simulink model "CSE1_CV3_1Straight"  (Simulink 7.3)
settings: Solver=ode4  StartTime=0.0  StopTime=inf  FixedStep=0.1  RelTol=1e-3
undefined symbols (not defined in the file or in its folder): eta1_0_real, v1_0_real, velocitySatValues1
libraries: simulink x68, dspmtrx3 x24, simulink_extras x23, marine_gnc x5, dspindex x5, dspinverses x4
(part 4 of 6)

== system CSE1_CV3_1Straight/Guidance Systems/Path-following/Line-Of-Sight/Dynamic assigment for sdot ==
  Delta : Inport
  epsilon_n^q : Inport  Port=2
  epsilon_n^s : Inport  Port=3
  epsilon_n : Inport  Port=4
  v_s : Inport  Port=5
  v_s^s : Inport  Port=6
  omega_s : Inport  Port=7
  omega_s^q : Inport  Port=8
  omega_s^s : Inport  Port=9
  v_s^t : Inport  Port=10
  f_s eq : Subsystem
  f_s^q eq : Subsystem
  f_s^s eq : Subsystem
  f_t eq : Subsystem
  f_s : Outport
  f_s^q : Outport  Port=2
  f_s^s : Outport  Port=3
  f_s^t : Outport  Port=4
  wires:
  Delta/1 -> f_s eq/1(Delta), f_s^q eq/1(Delta), f_s^s eq/1(Delta), f_t eq/1(Delta)
  epsilon_n/1 -> f_s eq/2(epsilon_n), f_s^q eq/2(epsilon_n), f_s^s eq/2(epsilon_n), f_t eq/2(epsilon_n)
  v_s/1 -> f_s eq/3(v_s), f_s^q eq/3(v_s), f_s^s eq/3(v_s)
  omega_s/1 -> f_s eq/4(omega_s)
  f_s eq/1(f_s) -> f_s/1
  f_s^q eq/1(f_s^q) -> f_s^q/1
  omega_s^q/1 -> f_s^q eq/4(omega_s^q)
  epsilon_n^q/1 -> f_s^q eq/5(epsilon_n^q)
  f_s^s eq/1(f_s^s) -> f_s^s/1
  omega_s^s/1 -> f_s^s eq/4(omega_s^s)
  epsilon_n^s/1 -> f_s^s eq/5(epsilon_n^s)
  v_s^s/1 -> f_s^s eq/6(v_s^s)
  f_t eq/1(f_t) -> f_s^t/1
  v_s^t/1 -> f_t eq/3(v_s^t)

== system CSE1_CV3_1Straight/Guidance Systems/Path-following/Line-Of-Sight/Gradient update law for sdot ==
  p_d^s^2 : Inport
  p_d^s : Inport  Port=2
  p_d : Inport  Port=3
  q : Inport  Port=4
  my : Inport  Port=5
  |p_d^s| : Inport  Port=6
  Subtract : Sum  Inputs=+-  OutDataType=fixdt(1, 16)  OutScaling=2^-10
  omega_s eq : Subsystem
  omega_s^q eq : Subsystem
  omega_s^s eq : Subsystem
  omega_s : Outport
  omega_s^q : Outport  Port=2
  omega_s^s : Outport  Port=3
  wires:
  p_d^s/1 -> omega_s eq/1(p_d^s), omega_s^q eq/1(p_d^s), omega_s^s eq/1(p_d^s)
  my/1 -> omega_s eq/3(my), omega_s^q eq/2(my), omega_s^s eq/3(my)
  |p_d^s|/1 -> omega_s eq/4(|p_d^s|), omega_s^q eq/3(|p_d^s|), omega_s^s eq/4(|p_d^s|)
  omega_s eq/1(omega_s) -> omega_s/1
  omega_s^q eq/1(omega_s^q) -> omega_s^q/1
  omega_s^s eq/1(omega_s^s) -> omega_s^s/1
  q/1 -> Subtract/1
  p_d/1 -> Subtract/2
  Subtract/1 -> omega_s eq/2(q - p_d), omega_s^s eq/2(q - p_d)
  p_d^s^2/1 -> omega_s^s eq/5(p_d^s^2)

== system CSE1_CV3_1Straight/Guidance Systems/Path-following/Line-Of-Sight/LOS heading ==
  psi_d : Inport
  psi_d^s : Inport  Port=2
  epsilon_n^qs : Inport  Port=3
  epsilon_n^q^2 : Inport  Port=4
  epsilon_n^s^2 : Inport  Port=5
  epsilon_n^q : Inport  Port=6
  epsilon_n^s : Inport  Port=7
  epsilon_n : Inport  Port=8
  psi_d¨^s^2 : Inport  Port=9
  Delta : Inport  Port=10
  psi_los eq : Subsystem
  psi_los^q eq : Subsystem
  psi_los^q^2 eq : Subsystem
  psi_los^qs = psi_los^sq : Subsystem
  psi_los^s eq : Subsystem
  psi_los^s^2 eq : Subsystem
  psi_los^q : Outport
  psi_los^s : Outport  Port=2
  psi_los : Outport  Port=3
  psi_los^qs : Outport  Port=4
  psi_los^q^2 : Outport  Port=5
  psi_los^s^2 : Outport  Port=6
  wires:
  psi_los eq/1(psi_los) -> psi_los/1
  psi_d/1 -> psi_los eq/1(psi_d)
  epsilon_n/1 -> psi_los eq/2(epsilon_n), psi_los^q eq/1(epsilon_n), psi_los^s eq/1(epsilon_n), psi_los^qs = psi_los^sq/1(epsilon_n), psi_los^q^2 eq/1(epsilon_n), psi_los^s^2 eq/1(epsilon_n)
  Delta/1 -> psi_los eq/3(Delta), psi_los^q eq/2(Delta), psi_los^s eq/2(Delta), psi_los^qs = psi_los^sq/2(Delta), psi_los^q^2 eq/2(Delta), psi_los^s^2 eq/2(Delta)
  epsilon_n^q/1 -> psi_los^q eq/3(epsilon_n^q), psi_los^qs = psi_los^sq/4(epsilon_n^q), psi_los^q^2 eq/3(epsilon_n^q)
  psi_los^q eq/1(psi_los^q) -> psi_los^q/1
  psi_los^s eq/1(psi_los^s) -> psi_los^s/1
  psi_d^s/1 -> psi_los^s eq/3(psi_d^s)
  psi_los^qs = psi_los^sq/1(psi_los^qs) -> psi_los^qs/1
  epsilon_n^s/1 -> psi_los^s eq/4(epsilon_n^s), psi_los^qs = psi_los^sq/3(epsilon_n^s), psi_los^s^2 eq/3(epsilon_n^s)
  epsilon_n^qs/1 -> psi_los^qs = psi_los^sq/5(epsilon_n^qs)
  psi_los^q^2 eq/1(psi_los^q^2) -> psi_los^q^2/1
  epsilon_n^q^2/1 -> psi_los^q^2 eq/4(epsilon_n^q^2)
  psi_d¨^s^2/1 -> psi_los^s^2 eq/4(psi_d¨^s^2)
  epsilon_n^s^2/1 -> psi_los^s^2 eq/5(epsilon_n^s^2)
  psi_los^s^2 eq/1(psi_los^s^2) -> psi_los^s^2/1

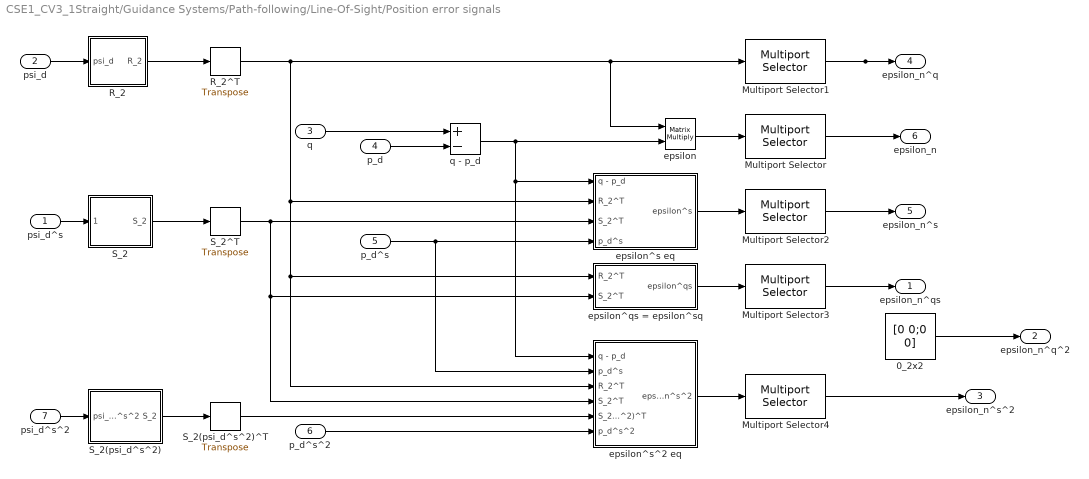
== system CSE1_CV3_1Straight/Guidance Systems/Path-following/Line-Of-Sight/Position error signals ==
  psi_d^s : Inport
  psi_d : Inport  Port=2
  q : Inport  Port=3
  p_d : Inport  Port=4
  p_d^s : Inport  Port=5
  p_d^s^2 : Inport  Port=6
  psi_d^s^2 : Inport  Port=7
  0_2x2 : Constant  Value=[0 0;0 0]  OutDataType=fixdt(1, 16)  OutScaling=2^0
  Multiport Selector{,1..4} (5 alike) : dspindex/Multiport Selector  rowsOrCols=Rows  idxCellArray={2}  idxErrMode=Clip Index
  R_2 : Subsystem  TreatAsAtomicUnit=on
      settings: MinAlgLoopOccurrences=on
  R_2^T : dspmtrx3/Transpose  SystemSampleTime=-1  Hermitian=off  overflowFlag=off
  S_2 : Subsystem  TreatAsAtomicUnit=on
      settings: MinAlgLoopOccurrences=on
  S_2(psi_d^s^2) : Subsystem  TreatAsAtomicUnit=on
      settings: MinAlgLoopOccurrences=on
  S_2(psi_d^s^2)^T : dspmtrx3/Transpose  SystemSampleTime=-1  Hermitian=off  overflowFlag=off
  S_2^T : dspmtrx3/Transpose  SystemSampleTime=-1  Hermitian=off  overflowFlag=off
  epsilon : Product  Multiplication=Matrix(*)  OutDataType=fixdt(1, 16)  OutScaling=2^0  RndMeth=Zero
  epsilon^qs = epsilon^sq : Subsystem
  epsilon^s eq : Subsystem
  epsilon^s^2 eq : Subsystem
  q - p_d : Sum  Inputs=+-  OutDataType=fixdt(1, 16)  OutScaling=2^-10
  epsilon_n^qs : Outport
  epsilon_n^q^2 : Outport  Port=2
  epsilon_n^s^2 : Outport  Port=3
  epsilon_n^q : Outport  Port=4
  epsilon_n^s : Outport  Port=5
  epsilon_n : Outport  Port=6
  wires:
  R_2/1(R_2) -> R_2^T/1
  psi_d/1 -> R_2/1(psi_d)
  q/1 -> q - p_d/1
  p_d/1 -> q - p_d/2
  R_2^T/1 -> epsilon/1, Multiport Selector1/1, epsilon^s eq/2(R_2^T), epsilon^qs = epsilon^sq/1(R_2^T), epsilon^s^2 eq/3(R_2^T)
  q - p_d/1 -> epsilon/2, epsilon^s eq/1(q - p_d), epsilon^s^2 eq/1(q - p_d)
  psi_d^s/1 -> S_2/1(psi_d^s)
  S_2/1(S_2) -> S_2^T/1
  p_d^s/1 -> epsilon^s eq/4(p_d^s), epsilon^s^2 eq/2(p_d^s)
  epsilon^s eq/1(epsilon^s) -> Multiport Selector2/1
  S_2^T/1 -> epsilon^s eq/3(S_2^T), epsilon^qs = epsilon^sq/2(S_2^T), epsilon^s^2 eq/4(S_2^T)
  epsilon^qs = epsilon^sq/1(epsilon^qs) -> Multiport Selector3/1
  0_2x2/1 -> epsilon_n^q^2/1
  epsilon/1 -> Multiport Selector/1
  Multiport Selector/1 -> epsilon_n/1
  Multiport Selector1/1 -> epsilon_n^q/1
  Multiport Selector2/1 -> epsilon_n^s/1
  Multiport Selector3/1 -> epsilon_n^qs/1
  psi_d^s^2/1 -> S_2(psi_d^s^2)/1(psi_d^s^2)
  S_2(psi_d^s^2)/1(S_2) -> S_2(psi_d^s^2)^T/1
  epsilon^s^2 eq/1(epsilon^s^2) -> Multiport Selector4/1
  Multiport Selector4/1 -> epsilon_n^s^2/1
  S_2(psi_d^s^2)^T/1 -> epsilon^s^2 eq/5(S_2(psi_d^s^2)^T)
  p_d^s^2/1 -> epsilon^s^2 eq/6(p_d^s^2)

== system CSE1_CV3_1Straight/Guidance Systems/Path-following/Path/Straight path ==
  s : Inport
  x_1 : Inport  Port=2
  y1 : Inport  Port=3
  x_2 : Inport  Port=4
  y_2 : Inport  Port=5
  0_2x1 : Constant  Value=0  VectorParams1D=off  OutDataType=fixdt(1, 16)  OutScaling=2^0
  Mux1 : Mux  Inputs=2
  p_d eq : Subsystem
  p_d^s eq : Subsystem
  |p_d^s| eq : Subsystem
  p_d : Outport
  p_d^s : Outport  Port=2
  p_d^s^2 : Outport  Port=3
  p_d^s^3 : Outport  Port=4
  |p_d^s| : Outport  Port=5
  wires:
  p_d^s eq/1(p_d^s) -> p_d^s/1, |p_d^s| eq/1(p_d^s)
  |p_d^s| eq/1(|p_d^s|) -> |p_d^s|/1
  s/1 -> p_d eq/1(s)
  x_1/1 -> p_d eq/2(x_1), p_d^s eq/1(x_1)
  y1/1 -> p_d eq/3(y_1), p_d^s eq/2(y_1)
  x_2/1 -> p_d eq/4(x_2), p_d^s eq/3(x_2)
  y_2/1 -> p_d eq/5(y_2), p_d^s eq/4(y_2)
  0_2x1/1 -> Mux1/1, Mux1/2
  Mux1/1 -> p_d^s^2/1, p_d^s^3/1
  p_d eq/1(p_d) -> p_d/1

== system CSE1_CV3_1Straight/Guidance Systems/Path-following/Speed assigment/v_s eq ==
  |p_d^s| : Inport
  u_d : Inport  Port=2
  Divide : Product  Inputs=*/  OutDataType=fixdt(1, 16)  OutScaling=2^-10
  v_s : Outport
  wires:
  Divide/1 -> v_s/1
  u_d/1 -> Divide/1
  |p_d^s|/1 -> Divide/2

== system CSE1_CV3_1Straight/Guidance Systems/Path-following/Speed assigment/v_s^s eq ==
  |p_d^s| : Inport
  u_d : Inport  Port=2
  p_d^s : Inport  Port=3
  p_d^s^2 : Inport  Port=4
  Constant : Constant  Value=3  OutDataType=fixdt(1, 16)  OutScaling=2^0
  Divide : Product  Inputs=*/  OutDataType=fixdt(1, 16)  OutScaling=2^-10
  Gain : Gain  Gain=-1  ParameterDataType=fixdt(1, 16)  ParameterScaling=2^0  OutDataType=fixdt(1, 16)  OutScaling=2^0
  Product : Product  OutDataType=fixdt(1, 16)  OutScaling=2^0  RndMeth=Zero
  Product1 : Product  Multiplication=Matrix(*)  OutDataType=fixdt(1, 16)  OutScaling=2^0  RndMeth=Zero
  p_d^s^T : dspmtrx3/Transpose  SystemSampleTime=-1  Hermitian=off  overflowFlag=off
  |p_d^s|^3 : Math  Operator=pow  OutDataType=fixdt(1, 16)  OutScaling=2^0  SaturateOnIntegerOverflow=on
  v_s^s : Outport
  wires:
  Product/1 -> Gain/1
  p_d^s/1 -> p_d^s^T/1
  p_d^s^T/1 -> Product1/1
  p_d^s^2/1 -> Product1/2
  |p_d^s|/1 -> |p_d^s|^3/1
  Constant/1 -> |p_d^s|^3/2
  Product1/1 -> Divide/1
  |p_d^s|^3/1 -> Divide/2
  Divide/1 -> Product/1
  u_d/1 -> Product/2
  Gain/1 -> v_s^s/1

== system CSE1_CV3_1Straight/Guidance Systems/Path-following/Speed assigment/v_s^t eq ==
  |p_d^s| : Inport
  u_d^t : Inport  Port=2
  Divide : Product  Inputs=*/  OutDataType=fixdt(1, 16)  OutScaling=2^-10
  v_s^t : Outport
  wires:
  Divide/1 -> v_s^t/1
  u_d^t/1 -> Divide/1
  |p_d^s|/1 -> Divide/2

== system CSE1_CV3_1Straight/Plants/Linear Simulator/Linear Vessel Dynamics/D_L ==
  -N_r : Gain  Gain=-1  ParameterDataType=fixdt(1, 16)  ParameterScaling=2^0  OutDataType=fixdt(1, 16)  OutScaling=2^0
  -N_v : Gain  Gain=-1  ParameterDataType=fixdt(1, 16)  ParameterScaling=2^0  OutDataType=fixdt(1, 16)  OutScaling=2^0
  -X_u : Gain  Gain=-1  ParameterDataType=fixdt(1, 16)  ParameterScaling=2^0  OutDataType=fixdt(1, 16)  OutScaling=2^0
  -Y_v : Gain  Gain=-1  ParameterDataType=fixdt(1, 16)  ParameterScaling=2^0  OutDataType=fixdt(1, 16)  OutScaling=2^0
  -Y_vr : Gain  Gain=-1  ParameterDataType=fixdt(1, 16)  ParameterScaling=2^0  OutDataType=fixdt(1, 16)  OutScaling=2^0
  D_L_{12..13,21,31} (4 alike) : Constant  Value=0
  Linear Dampning matrix : Reshape  OutputDimensionality=Customize  OutputDimensions=[3,3]
  Mux : Mux  Inputs=9
  N_r : Constant  Value=-1.900
  N_v : Constant  Value=0.18140
  X_u : Constant  Value=-0.59739
  Y_r : Constant  Value=-7.250
  Y_v : Constant  Value=-3.50625
  D_L : Outport
  wires:
  X_u/1 -> -X_u/1
  Mux/1 -> Linear Dampning matrix/1
  Linear Dampning matrix/1 -> D_L/1
  Y_v/1 -> -Y_v/1
  N_v/1 -> -N_v/1
  Y_r/1 -> -Y_vr/1
  N_r/1 -> -N_r/1
  -X_u/1 -> Mux/1
  D_L_21/1 -> Mux/2
  D_L_31/1 -> Mux/3
  D_L_12/1 -> Mux/4
  -Y_v/1 -> Mux/5
  -N_v/1 -> Mux/6
  D_L_13/1 -> Mux/7
  -Y_vr/1 -> Mux/8
  -N_r/1 -> Mux/9

== system CSE1_CV3_1Straight/Plants/Linear Simulator/Linear Vessel Dynamics/Initial eta ==
  Mux : Mux  Inputs=3
  psi_0 : Constant  Value=0  OutDataType=fixdt(1, 16)  OutScaling=2^0
  x_0 : Constant  Value=0  OutDataType=fixdt(1, 16)  OutScaling=2^0
  y_0 : Constant  Value=0  OutDataType=fixdt(1, 16)  OutScaling=2^0
  eta_0 : Outport  OutDataType=fixdt(1, 16)  OutScaling=2^0
  wires:
  x_0/1 -> Mux/1
  y_0/1 -> Mux/2
  psi_0/1 -> Mux/3
  Mux/1 -> eta_0/1

== system CSE1_CV3_1Straight/Plants/Linear Simulator/Linear Vessel Dynamics/Initial nu ==
  Mux : Mux  Inputs=3
  r_0 : Constant  Value=0  OutDataType=fixdt(1, 16)  OutScaling=2^0
  u_0 : Constant  Value=0  OutDataType=fixdt(1, 16)  OutScaling=2^0
  v_0 : Constant  Value=0  OutDataType=fixdt(1, 16)  OutScaling=2^0
  nu_0 : Outport  OutDataType=fixdt(1, 16)  OutScaling=2^0
  wires:
  u_0/1 -> Mux/1
  v_0/1 -> Mux/2
  r_0/1 -> Mux/3
  Mux/1 -> nu_0/1

== system CSE1_CV3_1Straight/Plants/Linear Simulator/Linear Vessel Dynamics/M_inv ==
  I_z : Constant  Value=1.760
  Inverse : Product  Inputs=/  Multiplication=Matrix(*)
  M : Reshape  OutputDimensionality=Customize  OutputDimensions=[3,3]
  M_{11,22..23,32..33} (5 alike) : Sum  Inputs=+-
  M_{12..13,21,31} (4 alike) : Constant  Value=0
  Mux : Mux  Inputs=9
  N_rdot : Constant  Value=-1.0
  N_vdot : Constant  Value=-0.0
  X_udot : Constant  Value=-2.0
  Y_rdot : Constant  Value=0.0
  Y_vdot : Constant  Value=-10.0
  m : Constant  Value=17.6
  m x_g : Product  RndMeth=Zero
  x_g : Constant  Value=0.03
  M_inv : Outport
  wires:
  m/1 -> M_11/1, M_22/1, m x_g/1
  X_udot/1 -> M_11/2
  Y_vdot/1 -> M_22/2
  x_g/1 -> m x_g/2
  m x_g/1 -> M_32/1, M_23/1
  N_vdot/1 -> M_32/2
  Y_rdot/1 -> M_23/2
  I_z/1 -> M_33/1
  N_rdot/1 -> M_33/2
  Inverse/1 -> M_inv/1
  M_11/1 -> Mux/1
  M_21/1 -> Mux/2
  M_31/1 -> Mux/3
  M_12/1 -> Mux/4
  M_22/1 -> Mux/5
  M_32/1 -> Mux/6
  M_13/1 -> Mux/7
  M_23/1 -> Mux/8
  M_33/1 -> Mux/9
  Mux/1 -> M/1
  M/1 -> Inverse/1

== system CSE1_CV3_1Straight/Plants/Linear Simulator/Linear Vessel Dynamics/R(psi) ==
  psi : Inport
  Mux : Mux  Inputs=9
  R(psi) : Reshape  OutputDimensionality=Customize  OutputDimensions=[3,3]
  R11 : Fcn  Expr=cos(u(1))
  R12 : Fcn  Expr=-1*sin(u(1))
  R{13,23,31..32} (4 alike) : Constant  Value=0
  R21 : Fcn  Expr=sin(u(1))
  R22 : Fcn  Expr=cos(u(1))
  R33 : Constant
  R : Outport
  wires:
  R(psi)/1 -> R/1
  Mux/1 -> R(psi)/1
  psi/1 -> R11/1, R21/1, R12/1, R22/1
  R11/1 -> Mux/1
  R21/1 -> Mux/2
  R31/1 -> Mux/3
  R12/1 -> Mux/4
  R22/1 -> Mux/5
  R32/1 -> Mux/6
  R13/1 -> Mux/7
  R33/1 -> Mux/9
  R23/1 -> Mux/8

== system CSE1_CV3_1Straight/Control Systems/DP control/Thruster allocation/f_act to u_act/f_1 to u_1 ==
  note: If < 0: control input is 1
      | if = 0 control input is 2
      | if > 0: control input is 3
  note: Check if the input value is less, equal or greater then zero
  note: The mapping is divided into 3 parts:
      | negative, zero and positive
  f_1 : Inport
  Gain : Gain  Gain=2  ParameterDataType=fixdt(1, 16)  ParameterScaling=2^0  OutDataType=fixdt(1, 16)  OutScaling=2^0
  Gain1 : Gain  Gain=3  ParameterDataType=fixdt(1, 16)  ParameterScaling=2^0  OutDataType=fixdt(1, 16)  OutScaling=2^0
  If < 0 : simulink/Logic and Bit Operations/Compare To Constant  SystemSampleTime=-1  relop=<  const=0  LogicOutDataTypeMode=uint8
  If > 0 : simulink/Logic and Bit Operations/Compare To Constant  SystemSampleTime=-1  relop=>  const=0  LogicOutDataTypeMode=uint8
  Multiport Switch : MultiPortSwitch  OutDataType=fixdt(1, 16)  OutScaling=2^0
  Sum : Sum  Inputs=+++  OutDataType=fixdt(1, 16)  OutScaling=2^0
  f_1 < 0 : Lookup  InputValues=|  Table=|  LookUpMeth=Interpolation-Use End Values  OutDataType=fixdt(1, 16)  OutScaling=2^0
      InputValues=|
      | [-1.324
      | -1.169
      | -0.919
      | -0.703
      | -0.535
      | -0.292
      | -0.165
      | -0.060
      | 0]
      Table=|
      | [-1.0000
      |    -0.9000
      |    -0.8000
      |    -0.7000
      |    -0.6000
      |    -0.5000
      |    -0.4000
      |    -0.3000
      |    -0.2089]
  f_1 = 0 : Constant  Value=0  OutDataType=fixdt(1, 16)  OutScaling=2^0
  f_1 > 0 : Lookup  InputValues=|  Table=|  LookUpMeth=Interpolation-Use End Values  OutDataType=fixdt(1, 16)  OutScaling=2^0
      InputValues=|
      | [0
      |     0.0510
      |     0.1530
      |     0.3080
      |     0.4800
      |     0.6630
      |     0.9110
      |     1.0570
      |     1.2210
      |     1.3740]
      Table=|
      | [0.0500
      |     0.1000
      |     0.2000
      |     0.3000
      |     0.4000
      |     0.5000
      |     0.6000
      |     0.7000
      |     0.8000
      |     0.9000]
  if == 0 : simulink/Logic and Bit Operations/Compare To Zero  SystemSampleTime=-1  relop===  LogicOutDataTypeMode=uint8
  u_1 : Outport
  wires:
  Multiport Switch/1 -> u_1/1
  Gain1/1 -> Sum/3
  Gain/1 -> Sum/2
  Sum/1 -> Multiport Switch/1
  If > 0/1 -> Gain1/1
  if == 0/1 -> Gain/1
  If < 0/1 -> Sum/1
  f_1/1 -> f_1 < 0/1, f_1 > 0/1, If < 0/1, if == 0/1, If > 0/1
  f_1 < 0/1 -> Multiport Switch/2
  f_1 = 0/1 -> Multiport Switch/3
  f_1 > 0/1 -> Multiport Switch/4

== system CSE1_CV3_1Straight/Control Systems/DP control/Thruster allocation/f_act to u_act/f_2 to u_2 ==
  note: If < 0: control input is 1
      | if = 0 control input is 2
      | if > 0: control input is 3
  note: Check if the input value is less, equal or greater then zero
  note: The mapping is divided into 3 parts:
      | Negative, zero and positive
  f_2 : Inport
  Gain : Gain  Gain=2  ParameterDataType=fixdt(1, 16)  ParameterScaling=2^0  OutDataType=fixdt(1, 16)  OutScaling=2^0
  Gain1 : Gain  Gain=3  ParameterDataType=fixdt(1, 16)  ParameterScaling=2^0  OutDataType=fixdt(1, 16)  OutScaling=2^0
  If < 0 : simulink/Logic and Bit Operations/Compare To Constant  SystemSampleTime=-1  relop=<  const=0  LogicOutDataTypeMode=uint8
  If > 0 : simulink/Logic and Bit Operations/Compare To Constant  SystemSampleTime=-1  relop=>  const=0  LogicOutDataTypeMode=uint8
  Multiport Switch : MultiPortSwitch  OutDataType=fixdt(1, 16)  OutScaling=2^0
  Sum : Sum  Inputs=+++  OutDataType=fixdt(1, 16)  OutScaling=2^0
  f_2 < 0 : Lookup  InputValues=|  Table=|  LookUpMeth=Interpolation-Use End Values  OutDataType=fixdt(1, 16)  OutScaling=2^0
      InputValues=|
      | [-0.766
      | -0.649
      | -0.522
      | -0.411
      | -0.323
      | -0.246
      | -0.156
      | -0.075
      | -0.018
      | -0.006
      | 0]
      Table=|
      | [-1.0000
      |    -0.9000
      |    -0.8000
      |    -0.7000
      |    -0.6000
      |    -0.5000
      |    -0.4000
      |    -0.3000
      |    -0.2000
      |    -0.1000
      |    -0.0466]
  f_2 = 0 : Constant  Value=0  OutDataType=fixdt(1, 16)  OutScaling=2^0
  f_2 > 0 : Lookup  InputValues=|  Table=|  LookUpMeth=Interpolation-Use End Values  OutDataType=fixdt(1, 16)  OutScaling=2^0
      InputValues=|
      | [0.000
      | 0.052
      | 0.207
      | 0.331
      | 0.509
      | 0.689
      | 0.829
      | 0.961
      | 1.079
      | 1.120
      | ]
      Table=|
      | [0.1665
      |     0.2000
      |     0.3000
      |     0.4000
      |     0.5000
      |     0.6000
      |     0.7000
      |     0.8000
      |     0.9000
      |     1.0000]
  if == 0 : simulink/Logic and Bit Operations/Compare To Zero  SystemSampleTime=-1  relop===  LogicOutDataTypeMode=uint8
  u_2 : Outport
  wires:
  f_2 > 0/1 -> Multiport Switch/4
  f_2 = 0/1 -> Multiport Switch/3
  f_2 < 0/1 -> Multiport Switch/2
  f_2/1 -> If > 0/1, if == 0/1, If < 0/1, f_2 > 0/1, f_2 < 0/1
  If < 0/1 -> Sum/1
  if == 0/1 -> Gain/1
  If > 0/1 -> Gain1/1
  Sum/1 -> Multiport Switch/1
  Gain/1 -> Sum/2
  Gain1/1 -> Sum/3
  Multiport Switch/1 -> u_2/1

== system CSE1_CV3_1Straight/Control Systems/DP control/Thruster allocation/f_act to u_act/f_3 to u_3 ==
  note: If < 0: control input is 1
      | if = 0 control input is 2
      | if > 0: control input is 3
  note: Check if the input value is less, equal or greater then zero
  note: The mapping is divided into 3 parts:
      | Negative, zero and positive
  f_3 : Inport
  Gain : Gain  Gain=2  ParameterDataType=fixdt(1, 16)  ParameterScaling=2^0  OutDataType=fixdt(1, 16)  OutScaling=2^0
  Gain1 : Gain  Gain=3  ParameterDataType=fixdt(1, 16)  ParameterScaling=2^0  OutDataType=fixdt(1, 16)  OutScaling=2^0
  If < 0 : simulink/Logic and Bit Operations/Compare To Constant  SystemSampleTime=-1  relop=<  const=0  LogicOutDataTypeMode=uint8
  If > 0 : simulink/Logic and Bit Operations/Compare To Constant  SystemSampleTime=-1  relop=>  const=0  LogicOutDataTypeMode=uint8
  Multiport Switch : MultiPortSwitch  OutDataType=fixdt(1, 16)  OutScaling=2^0
  Sum : Sum  Inputs=+++  OutDataType=fixdt(1, 16)  OutScaling=2^0
  f_3 < 0 : Lookup  InputValues=|  Table=|  LookUpMeth=Interpolation-Use End Values  OutDataType=fixdt(1, 16)  OutScaling=2^0
      InputValues=|
      | [-1.291
      | -1.088
      | -0.885
      | -0.618
      | -0.403
      | -0.211
      | -0.034
      | 0.000]
      Table=|
      | [-0.9000
      |    -0.8000
      |    -0.7000
      |    -0.6000
      |    -0.5000
      |    -0.4000
      |    -0.3000
      |    -0.2809]
  f_3 = 0 : Constant  Value=0  OutDataType=fixdt(1, 16)  OutScaling=2^0
  f_3 > 0 : Lookup  InputValues=|  Table=|  LookUpMeth=Interpolation-Use End Values  OutDataType=fixdt(1, 16)  OutScaling=2^0
      InputValues=|
      | [0.000
      | 0.014
      | 0.040
      | 0.147
      | 0.302
      | 0.494
      | 0.680
      | 0.968
      | 1.111
      | 1.289
      | 1.339]
      Table=|
      | [0.0452
      |     0.1000
      |     0.2000
      |     0.3000
      |     0.4000
      |     0.5000
      |     0.6000
      |     0.7000
      |     0.8000
      |     0.9000
      |     1.0000
      | ]
  if == 0 : simulink/Logic and Bit Operations/Compare To Zero  SystemSampleTime=-1  relop===  LogicOutDataTypeMode=uint8
  u_3 : Outport
  wires:
  Multiport Switch/1 -> u_3/1
  Gain1/1 -> Sum/3
  Gain/1 -> Sum/2
  Sum/1 -> Multiport Switch/1
  If > 0/1 -> Gain1/1
  if == 0/1 -> Gain/1
  If < 0/1 -> Sum/1
  f_3/1 -> f_3 < 0/1, f_3 > 0/1, If < 0/1, if == 0/1, If > 0/1
  f_3 < 0/1 -> Multiport Switch/2
  f_3 = 0/1 -> Multiport Switch/3
  f_3 > 0/1 -> Multiport Switch/4

== system CSE1_CV3_1Straight/Control Systems/DP control/Thruster allocation/f_act to u_act/f_4 to u_4 ==
  note: If < 0: control input is 1
      | if = 0 control input is 2
      | if > 0: control input is 3
  note: Check if the input value is less, equal or greater then zero
  note: The mapping is divided into 3 parts:
      | Negative, zero and positive
  f_4 : Inport
  Gain : Gain  Gain=2  ParameterDataType=fixdt(1, 16)  ParameterScaling=2^0  OutDataType=fixdt(1, 16)  OutScaling=2^0
  Gain1 : Gain  Gain=3  ParameterDataType=fixdt(1, 16)  ParameterScaling=2^0  OutDataType=fixdt(1, 16)  OutScaling=2^0
  If < 0 : simulink/Logic and Bit Operations/Compare To Constant  SystemSampleTime=-1  relop=<  const=0  LogicOutDataTypeMode=uint8
  If > 0 : simulink/Logic and Bit Operations/Compare To Constant  SystemSampleTime=-1  relop=>  const=0  LogicOutDataTypeMode=uint8
  Multiport Switch : MultiPortSwitch  OutDataType=fixdt(1, 16)  OutScaling=2^0
  Sum : Sum  Inputs=+++  OutDataType=fixdt(1, 16)  OutScaling=2^0
  f_4 < 0 : Lookup  InputValues=|  Table=|  LookUpMeth=Interpolation-Use End Values  OutDataType=fixdt(1, 16)  OutScaling=2^0
      InputValues=|
      | [-1.249
      | -1.225
      | -1.094
      | -0.896
      | -0.696
      | -0.502
      | -0.314
      | -0.169
      | -0.042
      | 0.000]
      Table=|
      | [-0.9000
      |    -0.8000
      |    -0.7000
      |    -0.6000
      |    -0.5000
      |    -0.4000
      |    -0.3000
      |    -0.2000
      |    -0.1000
      |    -0.0674]
  f_4 = 0 : Constant  Value=0  OutDataType=fixdt(1, 16)  OutScaling=2^0
  f_4 > 0 : Lookup  InputValues=|  Table=|  LookUpMeth=Interpolation-Use End Values  OutDataType=fixdt(1, 16)  OutScaling=2^0
      InputValues=|
      | [0.000
      | 0.063
      | 0.107
      | 0.274
      | 0.441
      | 0.599
      | 0.731]
      Table=|
      | [0.3588
      |     0.5000
      |     0.6000
      |     0.7000
      |     0.8000
      |     0.9000
      |     1.0000]
  if == 0 : simulink/Logic and Bit Operations/Compare To Zero  SystemSampleTime=-1  relop===  LogicOutDataTypeMode=uint8
  u_4 : Outport
  wires:
  f_4 > 0/1 -> Multiport Switch/4
  f_4 = 0/1 -> Multiport Switch/3
  f_4 < 0/1 -> Multiport Switch/2
  f_4/1 -> If > 0/1, if == 0/1, If < 0/1, f_4 > 0/1, f_4 < 0/1
  If < 0/1 -> Sum/1
  if == 0/1 -> Gain/1
  If > 0/1 -> Gain1/1
  Sum/1 -> Multiport Switch/1
  Gain/1 -> Sum/2
  Gain1/1 -> Sum/3
  Multiport Switch/1 -> u_4/1

== system CSE1_CV3_1Straight/Control Systems/DP control/Thruster allocation/f_act to u_act/f_5 to u_5 ==
  note: The mapping is divided into 3 parts:
      | Negative, zero and positive
  note: Check if the input value is less, equal or greater then zero
  note: If < 0: control input is 1
      | if = 0 control input is 2
      | if > 0: control input is 3
  f_5 : Inport
  Gain : Gain  Gain=2  ParameterDataType=fixdt(1, 16)  ParameterScaling=2^0  OutDataType=fixdt(1, 16)  OutScaling=2^0
  Gain1 : Gain  Gain=3  ParameterDataType=fixdt(1, 16)  ParameterScaling=2^0  OutDataType=fixdt(1, 16)  OutScaling=2^0
  If < 0 : simulink/Logic and Bit Operations/Compare To Constant  SystemSampleTime=-1  relop=<  const=0  LogicOutDataTypeMode=uint8
  If > 0 : simulink/Logic and Bit Operations/Compare To Constant  SystemSampleTime=-1  relop=>  const=0  LogicOutDataTypeMode=uint8
  Multiport Switch : MultiPortSwitch  OutDataType=fixdt(1, 16)  OutScaling=2^0
  Sum : Sum  Inputs=+++  OutDataType=fixdt(1, 16)  OutScaling=2^0
  f_5 < 0 : Lookup  InputValues=|  Table=|  LookUpMeth=Interpolation-Use End Values  OutDataType=fixdt(1, 16)  OutScaling=2^0
      InputValues=|
      | [-1.2630
      |    -1.0309
      |    -0.3808]
      Table=|
      | [-0.3000
      |    -0.2000
      |    -0.1000]
  f_5 = 0 : Constant  Value=0  OutDataType=fixdt(1, 16)  OutScaling=2^0
  f_5 > 0 : Lookup  InputValues=|  Table=|  LookUpMeth=Interpolation-Use End Values  OutDataType=fixdt(1, 16)  OutScaling=2^0
      InputValues=|
      | [0.3480
      |     0.8290
      |     1.0930]
      Table=|
      | [0.1000
      |     0.2000
      |     0.3000]
  if == 0 : simulink/Logic and Bit Operations/Compare To Zero  SystemSampleTime=-1  relop===  LogicOutDataTypeMode=uint8
  u_5 : Outport
  wires:
  Multiport Switch/1 -> u_5/1
  Gain1/1 -> Sum/3
  Gain/1 -> Sum/2
  Sum/1 -> Multiport Switch/1
  If > 0/1 -> Gain1/1
  if == 0/1 -> Gain/1
  If < 0/1 -> Sum/1
  f_5/1 -> f_5 < 0/1, f_5 > 0/1, If < 0/1, if == 0/1, If > 0/1
  f_5 < 0/1 -> Multiport Switch/2
  f_5 = 0/1 -> Multiport Switch/3
  f_5 > 0/1 -> Multiport Switch/4

== system CSE1_CV3_1Straight/Control Systems/DP control/Thruster allocation/tau to f_act/T_e ==
  -l_x1 : Gain  Gain=-1
  -l_x2 : Gain  Gain=-1
  -l_y2 : Gain  Gain=-1
  3x5 : Reshape  OutputDimensionality=Customize  OutputDimensions=[3,5]
  Mux : Mux  Inputs=15
  T_e{11,13,22,24..25} (5 alike) : Constant
  T_e{12,14..15,21,23} (5 alike) : Constant  Value=0
  l_x1 : Constant  Value=0.45
  l_x2 : Constant  Value=0.45
  l_x3 : Constant  Value=0.385
  l_y1 : Constant  Value=0.055
  l_y2 : Constant  Value=0.055
  T_e : Outport
  wires:
  l_x3/1 -> Mux/15
  T_e25/1 -> Mux/14
  T_e15/1 -> Mux/13
  -l_x2/1 -> Mux/12
  -l_y2/1 -> Mux/9
  -l_x1/1 -> Mux/6
  l_x2/1 -> -l_x2/1
  T_e24/1 -> Mux/11
  T_e14/1 -> Mux/10
  l_y2/1 -> -l_y2/1
  T_e23/1 -> Mux/8
  T_e13/1 -> Mux/7
  l_x1/1 -> -l_x1/1
  T_e22/1 -> Mux/5
  T_e12/1 -> Mux/4
  l_y1/1 -> Mux/3
  T_e21/1 -> Mux/2
  T_e11/1 -> Mux/1
  3x5/1 -> T_e/1
  Mux/1 -> 3x5/1

== system CSE1_CV3_1Straight/Control Systems/LgV design 2/Thruster allocation/f_act to u_act/f_1 to u_1 ==
  note: If < 0: control input is 1
      | if = 0 control input is 2
      | if > 0: control input is 3
  note: Check if the input value is less, equal or greater then zero
  note: The mapping is divided into 3 parts:
      | negative, zero and positive
  f_1 : Inport
  Gain : Gain  Gain=2  ParameterDataType=fixdt(1, 16)  ParameterScaling=2^0  OutDataType=fixdt(1, 16)  OutScaling=2^0
  Gain1 : Gain  Gain=3  ParameterDataType=fixdt(1, 16)  ParameterScaling=2^0  OutDataType=fixdt(1, 16)  OutScaling=2^0
  If < 0 : simulink/Logic and Bit Operations/Compare To Constant  SystemSampleTime=-1  relop=<  const=0  LogicOutDataTypeMode=uint8
  If > 0 : simulink/Logic and Bit Operations/Compare To Constant  SystemSampleTime=-1  relop=>  const=0  LogicOutDataTypeMode=uint8
  Multiport Switch : MultiPortSwitch  OutDataType=fixdt(1, 16)  OutScaling=2^0
  Sum : Sum  Inputs=+++  OutDataType=fixdt(1, 16)  OutScaling=2^0
  f_1 < 0 : Lookup  InputValues=|  Table=|  LookUpMeth=Interpolation-Use End Values  OutDataType=fixdt(1, 16)  OutScaling=2^0
      InputValues=|
      | [-1.324
      | -1.169
      | -0.919
      | -0.703
      | -0.535
      | -0.292
      | -0.165
      | -0.060
      | 0]
      Table=|
      | [-1.0000
      |    -0.9000
      |    -0.8000
      |    -0.7000
      |    -0.6000
      |    -0.5000
      |    -0.4000
      |    -0.3000
      |    -0.2089]
  f_1 = 0 : Constant  Value=0  OutDataType=fixdt(1, 16)  OutScaling=2^0
  f_1 > 0 : Lookup  InputValues=|  Table=|  LookUpMeth=Interpolation-Use End Values  OutDataType=fixdt(1, 16)  OutScaling=2^0
      InputValues=|
      | [0
      |     0.0510
      |     0.1530
      |     0.3080
      |     0.4800
      |     0.6630
      |     0.9110
      |     1.0570
      |     1.2210
      |     1.3740]
      Table=|
      | [0.0500
      |     0.1000
      |     0.2000
      |     0.3000
      |     0.4000
      |     0.5000
      |     0.6000
      |     0.7000
      |     0.8000
      |     0.9000]
  if == 0 : simulink/Logic and Bit Operations/Compare To Zero  SystemSampleTime=-1  relop===  LogicOutDataTypeMode=uint8
  u_1 : Outport
  wires:
  Multiport Switch/1 -> u_1/1
  Gain1/1 -> Sum/3
  Gain/1 -> Sum/2
  Sum/1 -> Multiport Switch/1
  If > 0/1 -> Gain1/1
  if == 0/1 -> Gain/1
  If < 0/1 -> Sum/1
  f_1/1 -> f_1 < 0/1, f_1 > 0/1, If < 0/1, if == 0/1, If > 0/1
  f_1 < 0/1 -> Multiport Switch/2
  f_1 = 0/1 -> Multiport Switch/3
  f_1 > 0/1 -> Multiport Switch/4

== system CSE1_CV3_1Straight/Control Systems/LgV design 2/Thruster allocation/f_act to u_act/f_2 to u_2 ==
  note: If < 0: control input is 1
      | if = 0 control input is 2
      | if > 0: control input is 3
  note: Check if the input value is less, equal or greater then zero
  note: The mapping is divided into 3 parts:
      | Negative, zero and positive
  f_2 : Inport
  Gain : Gain  Gain=2  ParameterDataType=fixdt(1, 16)  ParameterScaling=2^0  OutDataType=fixdt(1, 16)  OutScaling=2^0
  Gain1 : Gain  Gain=3  ParameterDataType=fixdt(1, 16)  ParameterScaling=2^0  OutDataType=fixdt(1, 16)  OutScaling=2^0
  If < 0 : simulink/Logic and Bit Operations/Compare To Constant  SystemSampleTime=-1  relop=<  const=0  LogicOutDataTypeMode=uint8
  If > 0 : simulink/Logic and Bit Operations/Compare To Constant  SystemSampleTime=-1  relop=>  const=0  LogicOutDataTypeMode=uint8
  Multiport Switch : MultiPortSwitch  OutDataType=fixdt(1, 16)  OutScaling=2^0
  Sum : Sum  Inputs=+++  OutDataType=fixdt(1, 16)  OutScaling=2^0
  f_2 < 0 : Lookup  InputValues=|  Table=|  LookUpMeth=Interpolation-Use End Values  OutDataType=fixdt(1, 16)  OutScaling=2^0
      InputValues=|
      | [-0.766
      | -0.649
      | -0.522
      | -0.411
      | -0.323
      | -0.246
      | -0.156
      | -0.075
      | -0.018
      | -0.006
      | 0]
      Table=|
      | [-1.0000
      |    -0.9000
      |    -0.8000
      |    -0.7000
      |    -0.6000
      |    -0.5000
      |    -0.4000
      |    -0.3000
      |    -0.2000
      |    -0.1000
      |    -0.0466]
  f_2 = 0 : Constant  Value=0  OutDataType=fixdt(1, 16)  OutScaling=2^0
  f_2 > 0 : Lookup  InputValues=|  Table=|  LookUpMeth=Interpolation-Use End Values  OutDataType=fixdt(1, 16)  OutScaling=2^0
      InputValues=|
      | [0.000
      | 0.052
      | 0.207
      | 0.331
      | 0.509
      | 0.689
      | 0.829
      | 0.961
      | 1.079
      | 1.120
      | ]
      Table=|
      | [0.1665
      |     0.2000
      |     0.3000
      |     0.4000
      |     0.5000
      |     0.6000
      |     0.7000
      |     0.8000
      |     0.9000
      |     1.0000]
  if == 0 : simulink/Logic and Bit Operations/Compare To Zero  SystemSampleTime=-1  relop===  LogicOutDataTypeMode=uint8
  u_2 : Outport
  wires:
  f_2 > 0/1 -> Multiport Switch/4
  f_2 = 0/1 -> Multiport Switch/3
  f_2 < 0/1 -> Multiport Switch/2
  f_2/1 -> If > 0/1, if == 0/1, If < 0/1, f_2 > 0/1, f_2 < 0/1
  If < 0/1 -> Sum/1
  if == 0/1 -> Gain/1
  If > 0/1 -> Gain1/1
  Sum/1 -> Multiport Switch/1
  Gain/1 -> Sum/2
  Gain1/1 -> Sum/3
  Multiport Switch/1 -> u_2/1

== system CSE1_CV3_1Straight/Control Systems/LgV design 2/Thruster allocation/f_act to u_act/f_3 to u_3 ==
  note: If < 0: control input is 1
      | if = 0 control input is 2
      | if > 0: control input is 3
  note: Check if the input value is less, equal or greater then zero
  note: The mapping is divided into 3 parts:
      | Negative, zero and positive
  f_3 : Inport
  Gain : Gain  Gain=2  ParameterDataType=fixdt(1, 16)  ParameterScaling=2^0  OutDataType=fixdt(1, 16)  OutScaling=2^0
  Gain1 : Gain  Gain=3  ParameterDataType=fixdt(1, 16)  ParameterScaling=2^0  OutDataType=fixdt(1, 16)  OutScaling=2^0
  If < 0 : simulink/Logic and Bit Operations/Compare To Constant  SystemSampleTime=-1  relop=<  const=0  LogicOutDataTypeMode=uint8
  If > 0 : simulink/Logic and Bit Operations/Compare To Constant  SystemSampleTime=-1  relop=>  const=0  LogicOutDataTypeMode=uint8
  Multiport Switch : MultiPortSwitch  OutDataType=fixdt(1, 16)  OutScaling=2^0
  Sum : Sum  Inputs=+++  OutDataType=fixdt(1, 16)  OutScaling=2^0
  f_3 < 0 : Lookup  InputValues=|  Table=|  LookUpMeth=Interpolation-Use End Values  OutDataType=fixdt(1, 16)  OutScaling=2^0
      InputValues=|
      | [-1.291
      | -1.088
      | -0.885
      | -0.618
      | -0.403
      | -0.211
      | -0.034
      | 0.000]
      Table=|
      | [-0.9000
      |    -0.8000
      |    -0.7000
      |    -0.6000
      |    -0.5000
      |    -0.4000
      |    -0.3000
      |    -0.2809]
  f_3 = 0 : Constant  Value=0  OutDataType=fixdt(1, 16)  OutScaling=2^0
  f_3 > 0 : Lookup  InputValues=|  Table=|  LookUpMeth=Interpolation-Use End Values  OutDataType=fixdt(1, 16)  OutScaling=2^0
      InputValues=|
      | [0.000
      | 0.014
      | 0.040
      | 0.147
      | 0.302
      | 0.494
      | 0.680
      | 0.968
      | 1.111
      | 1.289
      | 1.339]
      Table=|
      | [0.0452
      |     0.1000
      |     0.2000
      |     0.3000
      |     0.4000
      |     0.5000
      |     0.6000
      |     0.7000
      |     0.8000
      |     0.9000
      |     1.0000
      | ]
  if == 0 : simulink/Logic and Bit Operations/Compare To Zero  SystemSampleTime=-1  relop===  LogicOutDataTypeMode=uint8
  u_3 : Outport
  wires:
  Multiport Switch/1 -> u_3/1
  Gain1/1 -> Sum/3
  Gain/1 -> Sum/2
  Sum/1 -> Multiport Switch/1
  If > 0/1 -> Gain1/1
  if == 0/1 -> Gain/1
  If < 0/1 -> Sum/1
  f_3/1 -> f_3 < 0/1, f_3 > 0/1, If < 0/1, if == 0/1, If > 0/1
  f_3 < 0/1 -> Multiport Switch/2
  f_3 = 0/1 -> Multiport Switch/3
  f_3 > 0/1 -> Multiport Switch/4

== system CSE1_CV3_1Straight/Control Systems/LgV design 2/Thruster allocation/f_act to u_act/f_4 to u_4 ==
  note: If < 0: control input is 1
      | if = 0 control input is 2
      | if > 0: control input is 3
  note: Check if the input value is less, equal or greater then zero
  note: The mapping is divided into 3 parts:
      | Negative, zero and positive
  f_4 : Inport
  Gain : Gain  Gain=2  ParameterDataType=fixdt(1, 16)  ParameterScaling=2^0  OutDataType=fixdt(1, 16)  OutScaling=2^0
  Gain1 : Gain  Gain=3  ParameterDataType=fixdt(1, 16)  ParameterScaling=2^0  OutDataType=fixdt(1, 16)  OutScaling=2^0
  If < 0 : simulink/Logic and Bit Operations/Compare To Constant  SystemSampleTime=-1  relop=<  const=0  LogicOutDataTypeMode=uint8
  If > 0 : simulink/Logic and Bit Operations/Compare To Constant  SystemSampleTime=-1  relop=>  const=0  LogicOutDataTypeMode=uint8
  Multiport Switch : MultiPortSwitch  OutDataType=fixdt(1, 16)  OutScaling=2^0
  Sum : Sum  Inputs=+++  OutDataType=fixdt(1, 16)  OutScaling=2^0
  f_4 < 0 : Lookup  InputValues=|  Table=|  LookUpMeth=Interpolation-Use End Values  OutDataType=fixdt(1, 16)  OutScaling=2^0
      InputValues=|
      | [-1.249
      | -1.225
      | -1.094
      | -0.896
      | -0.696
      | -0.502
      | -0.314
      | -0.169
      | -0.042
      | 0.000]
      Table=|
      | [-0.9000
      |    -0.8000
      |    -0.7000
      |    -0.6000
      |    -0.5000
      |    -0.4000
      |    -0.3000
      |    -0.2000
      |    -0.1000
      |    -0.0674]
  f_4 = 0 : Constant  Value=0  OutDataType=fixdt(1, 16)  OutScaling=2^0
  f_4 > 0 : Lookup  InputValues=|  Table=|  LookUpMeth=Interpolation-Use End Values  OutDataType=fixdt(1, 16)  OutScaling=2^0
      InputValues=|
      | [0.000
      | 0.063
      | 0.107
      | 0.274
      | 0.441
      | 0.599
      | 0.731]
      Table=|
      | [0.3588
      |     0.5000
      |     0.6000
      |     0.7000
      |     0.8000
      |     0.9000
      |     1.0000]
  if == 0 : simulink/Logic and Bit Operations/Compare To Zero  SystemSampleTime=-1  relop===  LogicOutDataTypeMode=uint8
  u_4 : Outport
  wires:
  f_4 > 0/1 -> Multiport Switch/4
  f_4 = 0/1 -> Multiport Switch/3
  f_4 < 0/1 -> Multiport Switch/2
  f_4/1 -> If > 0/1, if == 0/1, If < 0/1, f_4 > 0/1, f_4 < 0/1
  If < 0/1 -> Sum/1
  if == 0/1 -> Gain/1
  If > 0/1 -> Gain1/1
  Sum/1 -> Multiport Switch/1
  Gain/1 -> Sum/2
  Gain1/1 -> Sum/3
  Multiport Switch/1 -> u_4/1

== system CSE1_CV3_1Straight/Control Systems/LgV design 2/Thruster allocation/f_act to u_act/f_5 to u_5 ==
  note: The mapping is divided into 3 parts:
      | Negative, zero and positive
  note: Check if the input value is less, equal or greater then zero
  note: If < 0: control input is 1
      | if = 0 control input is 2
      | if > 0: control input is 3
  f_5 : Inport
  Gain : Gain  Gain=2  ParameterDataType=fixdt(1, 16)  ParameterScaling=2^0  OutDataType=fixdt(1, 16)  OutScaling=2^0
  Gain1 : Gain  Gain=3  ParameterDataType=fixdt(1, 16)  ParameterScaling=2^0  OutDataType=fixdt(1, 16)  OutScaling=2^0
  If < 0 : simulink/Logic and Bit Operations/Compare To Constant  SystemSampleTime=-1  relop=<  const=0  LogicOutDataTypeMode=uint8
  If > 0 : simulink/Logic and Bit Operations/Compare To Constant  SystemSampleTime=-1  relop=>  const=0  LogicOutDataTypeMode=uint8
  Multiport Switch : MultiPortSwitch  OutDataType=fixdt(1, 16)  OutScaling=2^0
  Sum : Sum  Inputs=+++  OutDataType=fixdt(1, 16)  OutScaling=2^0
  f_5 < 0 : Lookup  InputValues=|  Table=|  LookUpMeth=Interpolation-Use End Values  OutDataType=fixdt(1, 16)  OutScaling=2^0
      InputValues=|
      | [-1.2630
      |    -1.0309
      |    -0.3808]
      Table=|
      | [-0.3000
      |    -0.2000
      |    -0.1000]
  f_5 = 0 : Constant  Value=0  OutDataType=fixdt(1, 16)  OutScaling=2^0
  f_5 > 0 : Lookup  InputValues=|  Table=|  LookUpMeth=Interpolation-Use End Values  OutDataType=fixdt(1, 16)  OutScaling=2^0
      InputValues=|
      | [0.3480
      |     0.8290
      |     1.0930]
      Table=|
      | [0.1000
      |     0.2000
      |     0.3000]
  if == 0 : simulink/Logic and Bit Operations/Compare To Zero  SystemSampleTime=-1  relop===  LogicOutDataTypeMode=uint8
  u_5 : Outport
  wires:
  Multiport Switch/1 -> u_5/1
  Gain1/1 -> Sum/3
  Gain/1 -> Sum/2
  Sum/1 -> Multiport Switch/1
  If > 0/1 -> Gain1/1
  if == 0/1 -> Gain/1
  If < 0/1 -> Sum/1
  f_5/1 -> f_5 < 0/1, f_5 > 0/1, If < 0/1, if == 0/1, If > 0/1
  f_5 < 0/1 -> Multiport Switch/2
  f_5 = 0/1 -> Multiport Switch/3
  f_5 > 0/1 -> Multiport Switch/4

== system CSE1_CV3_1Straight/Control Systems/LgV design 2/Thruster allocation/tau to f_act/T_e ==
  -l_x1 : Gain  Gain=-1
  -l_x2 : Gain  Gain=-1
  -l_y2 : Gain  Gain=-1
  3x5 : Reshape  OutputDimensionality=Customize  OutputDimensions=[3,5]
  Mux : Mux  Inputs=15
  T_e{11,13,22,24..25} (5 alike) : Constant
  T_e{12,14..15,21,23} (5 alike) : Constant  Value=0
  l_x1 : Constant  Value=0.45
  l_x2 : Constant  Value=0.45
  l_x3 : Constant  Value=0.385
  l_y1 : Constant  Value=0.055
  l_y2 : Constant  Value=0.055
  T_e : Outport
  wires:
  l_x3/1 -> Mux/15
  T_e25/1 -> Mux/14
  T_e15/1 -> Mux/13
  -l_x2/1 -> Mux/12
  -l_y2/1 -> Mux/9
  -l_x1/1 -> Mux/6
  l_x2/1 -> -l_x2/1
  T_e24/1 -> Mux/11
  T_e14/1 -> Mux/10
  l_y2/1 -> -l_y2/1
  T_e23/1 -> Mux/8
  T_e13/1 -> Mux/7
  l_x1/1 -> -l_x1/1
  T_e22/1 -> Mux/5
  T_e12/1 -> Mux/4
  l_y1/1 -> Mux/3
  T_e21/1 -> Mux/2
  T_e11/1 -> Mux/1
  3x5/1 -> T_e/1
  Mux/1 -> 3x5/1

== system CSE1_CV3_1Straight/Control Systems/LgV design 2/z_1 eq/heading to pipi/rad to pi2pi ==
  note: x
  note: r
  x (rad) : Inport  OutDataType=sfix(16)  OutScaling=2^0
  Constant : Constant  Value=2*180  OutDataType=sfix(16)  OutScaling=2^0
  Degrees to Radians : simulink_extras/Transformations/Degrees to Radians  SystemSampleTime=-1
  Gain : Gain  Gain=180  ParameterDataType=sfix(16)  ParameterScaling=2^0  OutDataType=sfix(16)  OutScaling=2^0  SaturateOnIntegerOverflow=on  OutDataTypeStr=Inherit: Same as input  ParamDataTypeStr=Inherit: Same as input
  Math Function : Math  Operator=rem  OutDataType=sfix(16)  OutScaling=2^0  SaturateOnIntegerOverflow=on
  Radians to Degrees : simulink_extras/Transformations/Radians to Degrees  SystemSampleTime=-1
  Saturation : Saturate  UpperLimit=1e10  LowerLimit=-1e10
  Sign : Signum
  Sum : Sum  Inputs=|+-  OutDataType=sfix(16)  OutScaling=2^0  SaturateOnIntegerOverflow=on
  Sum1 : Sum  Inputs=|++  OutDataType=sfix(16)  OutScaling=2^0  SaturateOnIntegerOverflow=on
  -pi to pi : Outport  OutDataType=sfix(16)  OutScaling=2^0
  wires:
  Saturation/1 -> Sum1/1, Sign/1
  x (rad)/1 -> Radians to Degrees/1
  Sign/1 -> Gain/1
  Gain/1 -> Sum/2, Sum1/2
  Sum1/1 -> Math Function/1
  Constant/1 -> Math Function/2
  Math Function/1 -> Sum/1
  Sum/1 -> Degrees to Radians/1
  Degrees to Radians/1 -> -pi to pi/1
  Radians to Degrees/1 -> Saturation/1

== system CSE1_CV3_1Straight/Control Systems/LgV design 2/z_1 eq/heading to pipi1/rad to pi2pi ==
  note: x
  note: r
  x (rad) : Inport  OutDataType=sfix(16)  OutScaling=2^0
  Constant : Constant  Value=2*180  OutDataType=sfix(16)  OutScaling=2^0
  Degrees to Radians : simulink_extras/Transformations/Degrees to Radians  SystemSampleTime=-1
  Gain : Gain  Gain=180  ParameterDataType=sfix(16)  ParameterScaling=2^0  OutDataType=sfix(16)  OutScaling=2^0  SaturateOnIntegerOverflow=on  OutDataTypeStr=Inherit: Same as input  ParamDataTypeStr=Inherit: Same as input
  Math Function : Math  Operator=rem  OutDataType=sfix(16)  OutScaling=2^0  SaturateOnIntegerOverflow=on
  Radians to Degrees : simulink_extras/Transformations/Radians to Degrees  SystemSampleTime=-1
  Saturation : Saturate  UpperLimit=1e10  LowerLimit=-1e10
  Sign : Signum
  Sum : Sum  Inputs=|+-  OutDataType=sfix(16)  OutScaling=2^0  SaturateOnIntegerOverflow=on
  Sum1 : Sum  Inputs=|++  OutDataType=sfix(16)  OutScaling=2^0  SaturateOnIntegerOverflow=on
  -pi to pi : Outport  OutDataType=sfix(16)  OutScaling=2^0
  wires:
  Saturation/1 -> Sum1/1, Sign/1
  x (rad)/1 -> Radians to Degrees/1
  Sign/1 -> Gain/1
  Gain/1 -> Sum/2, Sum1/2
  Sum1/1 -> Math Function/1
  Constant/1 -> Math Function/2
  Math Function/1 -> Sum/1
  Sum/1 -> Degrees to Radians/1
  Degrees to Radians/1 -> -pi to pi/1
  Radians to Degrees/1 -> Saturation/1

== system CSE1_CV3_1Straight/Control Systems/Manual Thruster control/Subsystem/f_act to tau/T_e ==
  -l_x1 : Gain  Gain=-1
  -l_x2 : Gain  Gain=-1
  -l_y2 : Gain  Gain=-1
  3x5 : Reshape  OutputDimensionality=Customize  OutputDimensions=[3,5]
  Mux : Mux  Inputs=15
  T_e{11,13,22,24..25} (5 alike) : Constant
  T_e{12,14..15,21,23} (5 alike) : Constant  Value=0
  l_x1 : Constant  Value=0.45
  l_x2 : Constant  Value=0.45
  l_x3 : Constant  Value=0.385
  l_y1 : Constant  Value=0.055
  l_y2 : Constant  Value=0.055
  T_e : Outport
  wires:
  Mux/1 -> 3x5/1
  3x5/1 -> T_e/1
  T_e11/1 -> Mux/1
  T_e21/1 -> Mux/2
  l_y1/1 -> Mux/3
  T_e12/1 -> Mux/4
  T_e22/1 -> Mux/5
  l_x1/1 -> -l_x1/1
  T_e13/1 -> Mux/7
  T_e23/1 -> Mux/8
  l_y2/1 -> -l_y2/1
  T_e14/1 -> Mux/10
  T_e24/1 -> Mux/11
  l_x2/1 -> -l_x2/1
  -l_x1/1 -> Mux/6
  -l_y2/1 -> Mux/9
  -l_x2/1 -> Mux/12
  T_e15/1 -> Mux/13
  T_e25/1 -> Mux/14
  l_x3/1 -> Mux/15

== system CSE1_CV3_1Straight/Control Systems/Nonlinear PID/Control law/tau_FF/M ==
  3x3 : Reshape  OutputDimensionality=Customize  OutputDimensions=[3,3]
  I_z : Constant  Value=1.760
  M_{11,22..23,32..33} (5 alike) : Sum  Inputs=+-
  M_{12..13,21,31} (4 alike) : Constant  Value=0
  Mux : Mux  Inputs=9
  N_rdot : Constant  Value=-1.0
  N_vdot : Constant  Value=-0.0
  X_udot : Constant  Value=-2.0
  Y_rdot : Constant  Value=0.0
  Y_vdot : Constant  Value=-10.0
  m : Constant  Value=17.6
  m x_g : Product  RndMeth=Zero
  x_g : Constant  Value=0.03
  M : Outport
  wires:
  3x3/1 -> M/1
  Mux/1 -> 3x3/1
  M_33/1 -> Mux/9
  M_23/1 -> Mux/8
  M_13/1 -> Mux/7
  M_32/1 -> Mux/6
  M_22/1 -> Mux/5
  M_12/1 -> Mux/4
  M_31/1 -> Mux/3
  M_21/1 -> Mux/2
  M_11/1 -> Mux/1
  N_rdot/1 -> M_33/2
  I_z/1 -> M_33/1
  Y_rdot/1 -> M_23/2
  N_vdot/1 -> M_32/2
  m x_g/1 -> M_23/1, M_32/1
  x_g/1 -> m x_g/2
  Y_vdot/1 -> M_22/2
  X_udot/1 -> M_11/2
  m/1 -> m x_g/1, M_22/1, M_11/1

== system CSE1_CV3_1Straight/Control Systems/Nonlinear PID/Control law/tau_FL/D_L ==
  -N_r : Gain  Gain=-1  ParameterDataType=fixdt(1, 16)  ParameterScaling=2^0  OutDataType=fixdt(1, 16)  OutScaling=2^0
  -N_v : Gain  Gain=-1  ParameterDataType=fixdt(1, 16)  ParameterScaling=2^0  OutDataType=fixdt(1, 16)  OutScaling=2^0
  -X_u : Gain  Gain=-1  ParameterDataType=fixdt(1, 16)  ParameterScaling=2^0  OutDataType=fixdt(1, 16)  OutScaling=2^0
  -Y_v : Gain  Gain=-1  ParameterDataType=fixdt(1, 16)  ParameterScaling=2^0  OutDataType=fixdt(1, 16)  OutScaling=2^0
  -Y_vr : Gain  Gain=-1  ParameterDataType=fixdt(1, 16)  ParameterScaling=2^0  OutDataType=fixdt(1, 16)  OutScaling=2^0
  D_L_{12..13,21,31} (4 alike) : Constant  Value=0
  Linear Dampning matrix : Reshape  OutputDimensionality=Customize  OutputDimensions=[3,3]
  Mux : Mux  Inputs=9
  N_r : Constant  Value=-1.900
  N_v : Constant  Value=0.18140
  X_u : Constant  Value=-0.59739
  Y_r : Constant  Value=-7.250
  Y_v : Constant  Value=-3.50625
  D_L : Outport
  wires:
  -N_r/1 -> Mux/9
  -Y_vr/1 -> Mux/8
  D_L_13/1 -> Mux/7
  -N_v/1 -> Mux/6
  -Y_v/1 -> Mux/5
  D_L_12/1 -> Mux/4
  D_L_31/1 -> Mux/3
  D_L_21/1 -> Mux/2
  -X_u/1 -> Mux/1
  N_r/1 -> -N_r/1
  Y_r/1 -> -Y_vr/1
  N_v/1 -> -N_v/1
  Y_v/1 -> -Y_v/1
  Linear Dampning matrix/1 -> D_L/1
  Mux/1 -> Linear Dampning matrix/1
  X_u/1 -> -X_u/1

== system CSE1_CV3_1Straight/Control Systems/Nonlinear PID/Error/heading to pipi/rad to pi2pi ==
  note: x
  note: r
  x (rad) : Inport  OutDataType=sfix(16)  OutScaling=2^0
  Constant : Constant  Value=2*180  OutDataType=sfix(16)  OutScaling=2^0
  Degrees to Radians : simulink_extras/Transformations/Degrees to Radians  SystemSampleTime=-1
  Gain : Gain  Gain=180  ParameterDataType=sfix(16)  ParameterScaling=2^0  OutDataType=sfix(16)  OutScaling=2^0  SaturateOnIntegerOverflow=on  OutDataTypeStr=Inherit: Same as input  ParamDataTypeStr=Inherit: Same as input
  Math Function : Math  Operator=rem  OutDataType=sfix(16)  OutScaling=2^0  SaturateOnIntegerOverflow=on
  Radians to Degrees : simulink_extras/Transformations/Radians to Degrees  SystemSampleTime=-1
  Saturation : Saturate  UpperLimit=1e10  LowerLimit=-1e10
  Sign : Signum
  Sum : Sum  Inputs=|+-  OutDataType=sfix(16)  OutScaling=2^0  SaturateOnIntegerOverflow=on
  Sum1 : Sum  Inputs=|++  OutDataType=sfix(16)  OutScaling=2^0  SaturateOnIntegerOverflow=on
  -pi to pi : Outport  OutDataType=sfix(16)  OutScaling=2^0
  wires:
  Saturation/1 -> Sum1/1, Sign/1
  x (rad)/1 -> Radians to Degrees/1
  Sign/1 -> Gain/1
  Gain/1 -> Sum/2, Sum1/2
  Sum1/1 -> Math Function/1
  Constant/1 -> Math Function/2
  Math Function/1 -> Sum/1
  Sum/1 -> Degrees to Radians/1
  Degrees to Radians/1 -> -pi to pi/1
  Radians to Degrees/1 -> Saturation/1

== system CSE1_CV3_1Straight/Control Systems/Nonlinear PID/Error/heading to pipi1/rad to pi2pi ==
  note: r
  note: x
  x (rad) : Inport  OutDataType=sfix(16)  OutScaling=2^0
  Constant : Constant  Value=2*180  OutDataType=sfix(16)  OutScaling=2^0
  Degrees to Radians : simulink_extras/Transformations/Degrees to Radians  SystemSampleTime=-1
  Gain : Gain  Gain=180  ParameterDataType=sfix(16)  ParameterScaling=2^0  OutDataType=sfix(16)  OutScaling=2^0  SaturateOnIntegerOverflow=on  OutDataTypeStr=Inherit: Same as input  ParamDataTypeStr=Inherit: Same as input
  Math Function : Math  Operator=rem  OutDataType=sfix(16)  OutScaling=2^0  SaturateOnIntegerOverflow=on
  Radians to Degrees : simulink_extras/Transformations/Radians to Degrees  SystemSampleTime=-1
  Saturation : Saturate  UpperLimit=1e10  LowerLimit=-1e10
  Sign : Signum
  Sum : Sum  Inputs=|+-  OutDataType=sfix(16)  OutScaling=2^0  SaturateOnIntegerOverflow=on
  Sum1 : Sum  Inputs=|++  OutDataType=sfix(16)  OutScaling=2^0  SaturateOnIntegerOverflow=on
  -pi to pi : Outport  OutDataType=sfix(16)  OutScaling=2^0
  wires:
  Radians to Degrees/1 -> Saturation/1
  Degrees to Radians/1 -> -pi to pi/1
  Sum/1 -> Degrees to Radians/1
  Math Function/1 -> Sum/1
  Constant/1 -> Math Function/2
  Sum1/1 -> Math Function/1
  Gain/1 -> Sum1/2, Sum/2
  Sign/1 -> Gain/1
  x (rad)/1 -> Radians to Degrees/1
  Saturation/1 -> Sign/1, Sum1/1
